simulink model "state_feedback"  (R2018a)
settings: Solver=VariableStepAuto  StartTime=0.0  StopTime=30  RelTol=1e-3
undefined symbols (not defined in the file): A, B, C, K, L
settings Model: Creator=Blake  LastModifiedBy=Blake

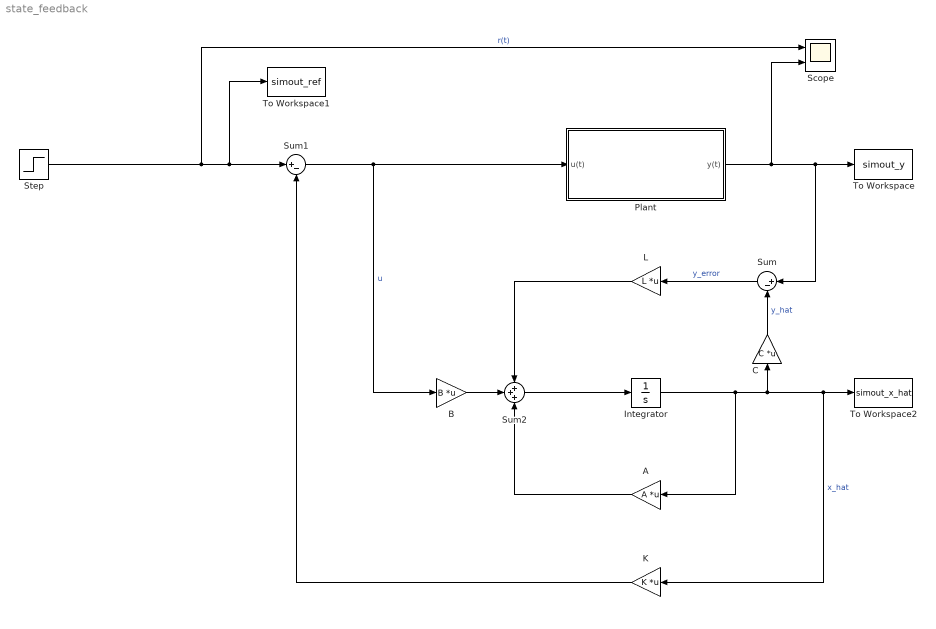
== system state_feedback ==
  A : Gain  Gain=A  Multiplication=Matrix(K*u)
  B : Gain  Gain=B  Multiplication=Matrix(K*u)
  C : Gain  Gain=C  Multiplication=Matrix(K*u)
  Integrator : Integrator
  K : Gain  Gain=K  Multiplication=Matrix(K*u)
  L : Gain  Gain=L  Multiplication=Matrix(K*u)
  Plant : Subsystem
  Scope : Scope  NumInputPorts=2
  Step : Step  SampleTime=0
  Sum : Sum  Inputs=|+-
  Sum1 : Sum  Inputs=|+-
  Sum2 : Sum  Inputs=+++
  To Workspace : ToWorkspace  VariableName=simout_y  SaveFormat=Timeseries  SampleTime=-1
  To Workspace1 : ToWorkspace  VariableName=simout_ref  SaveFormat=Timeseries  SampleTime=-1
  To Workspace2 : ToWorkspace  VariableName=simout_x_hat  SaveFormat=Timeseries  SampleTime=-1
  wires:
  Step/1 -> Scope/1, To Workspace1/1, Sum1/1  "r(t)"
  Sum1/1 -> B/1, Plant/1(u(t))  "u"
  Plant/1(y(t)) -> Scope/2, Sum/1, To Workspace/1
  C/1 -> Sum/2  "y_hat"
  Sum/1 -> L/1  "y_error"
  Integrator/1 -> A/1, K/1, To Workspace2/1, C/1  "x_hat"
  Sum2/1 -> Integrator/1
  L/1 -> Sum2/1
  A/1 -> Sum2/3
  B/1 -> Sum2/2
  K/1 -> Sum1/2

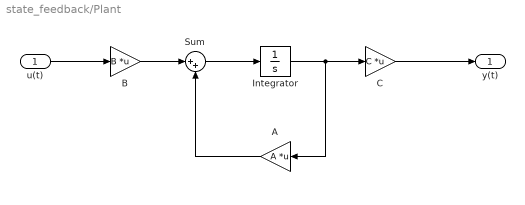
== system state_feedback/Plant ==
  u(t) : Inport
  A : Gain  Gain=A  Multiplication=Matrix(K*u)
  B : Gain  Gain=B  Multiplication=Matrix(K*u)
  C : Gain  Gain=C  Multiplication=Matrix(K*u)
  Integrator : Integrator
  Sum : Sum  Inputs=|++
  y(t) : Outport
  wires:
  A/1 -> Sum/2
  B/1 -> Sum/1
  C/1 -> y(t)/1
  Sum/1 -> Integrator/1
  Integrator/1 -> A/1, C/1
  u(t)/1 -> B/1
